simulink model "trajectory"  (R2021a)
settings: Solver=VariableStepAuto  StartTime=0.0  StopTime=10.0  RelTol=1e-3
libraries: robotcorelib x2
settings Model: Creator=ASUS  LastModifiedBy=ASUS

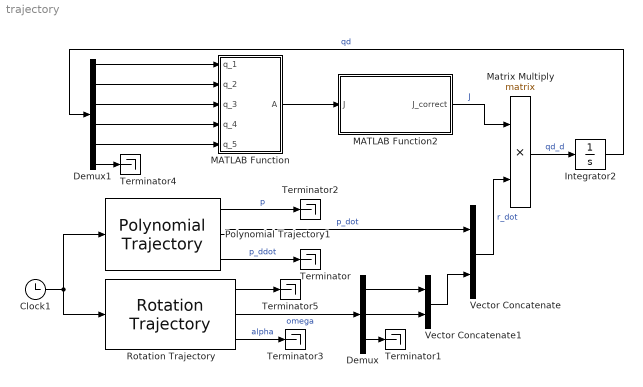
== system trajectory ==
  Clock1 : Clock
  Demux : Demux  Outputs=3
  Demux1 : Demux  Outputs=6
  Integrator2 : Integrator  InitialCondition=2
  MATLAB Function : MATLAB Function  TreatAsAtomicUnit=on
  MATLAB Function2 : MATLAB Function  TreatAsAtomicUnit=on
  Matrix Multiply : Product  Multiplication=Matrix(*)
  Polynomial Trajectory1 : robotcorelib/Polynomial Trajectory  WaypointSource=Internal  Waypoints=[ 0, 0.1, 0.1; 0, 0.2, 0.1; 0, 0.1, 0.1]  TimePoints=[ 0, 3, 5 ]  TimeInterval=[ 1, 4 ]  Method=Cubic Polynomial  ParameterSource=Internal  VelocityBoundaryCondition=zeros( 3, 3)  AccelerationBoundaryCondition=zeros( 2, 5 )  SimulateUsing=Interpreted execution
  Rotation Trajectory : robotcorelib/Rotation Trajectory  WaypointFormat=Quaternion  WaypointSource=Internal  R0=[ 1, 0, 0, 0 ]'  RF=[ 0.1, 0.2, 0.5, 0 ]'  TimeInterval=[ 0, 5 ]  CustomTimeScaling=off  ParameterSource=Internal  TSTime=0:0.1:1  TimeScaling=[ 0:0.1:1; ones( 1, 11 ); zeros( 1, 11 ) ]  SimulateUsing=Interpreted execution
      settings: SourceProductBaseCode=NV,RO,RR,UV
  Terminator{,1..5} (6 alike) : Terminator
  Vector Concatenate : Concatenate
  Vector Concatenate1 : Concatenate
  wires:
  Clock1/1 -> Polynomial Trajectory1/1, Rotation Trajectory/1
  Polynomial Trajectory1/3 -> Terminator/1  "p_ddot"
  Polynomial Trajectory1/2 -> Vector Concatenate/1  "p_dot"
  Polynomial Trajectory1/1 -> Terminator2/1  "p"
  Rotation Trajectory/1 -> Terminator5/1
  Rotation Trajectory/3 -> Terminator3/1  "alpha"
  MATLAB Function/1(A) -> MATLAB Function2/1(J)
  MATLAB Function2/1(J_correct) -> Matrix Multiply/1  "J"
  Demux/3 -> Terminator1/1
  Demux/1 -> Vector Concatenate1/1
  Demux/2 -> Vector Concatenate1/2
  Rotation Trajectory/2 -> Demux/1  "omega"
  Vector Concatenate1/1 -> Vector Concatenate/2
  Vector Concatenate/1 -> Matrix Multiply/2  "r_dot"
  Matrix Multiply/1 -> Integrator2/1  "qd_d"
  Integrator2/1 -> Demux1/1  "qd"
  Demux1/6 -> Terminator4/1
  Demux1/1 -> MATLAB Function/1(q_1)
  Demux1/2 -> MATLAB Function/2(q_2)
  Demux1/3 -> MATLAB Function/3(q_3)
  Demux1/4 -> MATLAB Function/4(q_4)
  Demux1/5 -> MATLAB Function/5(q_5)

== matlab function trajectory/MATLAB Function ==
  data: q_1 input; A output; q_2 input; q_3 input; q_4 input; q_5 input
function A = fcn(q_1,q_2,q_3,q_4,q_5)


A = reshape([cos(q_1).*(cos(q_5).*8.1141e-2-cos(q_1).*(cos(q_3).*(sin(q_4).*sin(q_5).*8.1141e-2-cos(q_4).*(cos(q_5).*4.968453296480769e-18-9.456e-2))+sin(q_3).*(cos(q_4).*sin(q_5).*8.1141e-2+sin(q_4).*(cos(q_5).*4.968453296480769e-18-9.456e-2)+3.9225e-1)).*6.123233995736766e-17-sin(q_2).*(cos(q_3).*(cos(q_4).*sin(q_5).*8.1141e-2+sin(q_4).*(cos(q_5).*4.968453296480769e-18-9.456e-2)+3.9225e-1)-sin(q_3).*(sin(q_4).*sin(q_5).*8.1141e-2-cos(q_4).*(cos(q_5).*4.968453296480769e-18-9.456e-2))+1.7e+1./4.0e+1).*6.123233995736766e-17+1.0915e-1)-sin(q_1).*(cos(q_2).*(cos(q_3).*(cos(q_4).*sin(q_5).*8.1141e-2+sin(q_4).*(cos(q_5).*4.968453296480769e-18-9.456e-2)+3.9225e-1)-sin(q_3).*(sin(q_4).*sin(q_5).*8.1141e-2-cos(q_4).*(cos(q_5).*4.968453296480769e-18-9.456e-2))+1.7e+1./4.0e+1)-sin(q_2).*(cos(q_3).*(sin(q_4).*sin(q_5).*8.1141e-2-cos(q_4).*(cos(q_5).*4.968453296480769e-18-9.456e-2))+sin(q_3).*(cos(q_4).*sin(q_5).*8.1141e-2+sin(q_4).*(cos(q_5).*4.968453296480769e-18-9.456e-2)+3.9225e-1)))+sin(q_1).^2.*(cos(q_3).*(sin(q_4).*sin(q_5).*8.1141e-2-cos(q_4).*(cos(q_5).*4.968453296480769e-18-9.456e-2))+sin(q_3).*(cos(q_4).*sin(q_5).*8.1141e-2+sin(q_4).*(cos(q_5).*4.968453296480769e-18-9.456e-2)+3.9225e-1)).*6.123233995736766e-17,sin(q_1).*(cos(q_5).*8.1141e-2-cos(q_1).*(cos(q_3).*(sin(q_4).*sin(q_5).*8.1141e-2-cos(q_4).*(cos(q_5).*4.968453296480769e-18-9.456e-2))+sin(q_3).*(cos(q_4).*sin(q_5).*8.1141e-2+sin(q_4).*(cos(q_5).*4.968453296480769e-18-9.456e-2)+3.9225e-1)).*6.123233995736766e-17-sin(q_2).*(cos(q_3).*(cos(q_4).*sin(q_5).*8.1141e-2+sin(q_4).*(cos(q_5).*4.968453296480769e-18-9.456e-2)+3.9225e-1)-sin(q_3).*(sin(q_4).*sin(q_5).*8.1141e-2-cos(q_4).*(cos(q_5).*4.968453296480769e-18-9.456e-2))+1.7e+1./4.0e+1).*6.123233995736766e-17+1.0915e-1)+cos(q_1).*(cos(q_2).*(cos(q_3).*(cos(q_4).*sin(q_5).*8.1141e-2+sin(q_4).*(cos(q_5).*4.968453296480769e-18-9.456e-2)+3.9225e-1)-sin(q_3).*(sin(q_4).*sin(q_5).*8.1141e-2-cos(q_4).*(cos(q_5).*4.968453296480769e-18-9.456e-2))+1.7e+1./4.0e+1)-sin(q_2).*(cos(q_3).*(sin(q_4).*sin(q_5).*8.1141e-2-cos(q_4).*(cos(q_5).*4.968453296480769e-18-9.456e-2))+sin(q_3).*(cos(q_4).*sin(q_5).*8.1141e-2+sin(q_4).*(cos(q_5).*4.968453296480769e-18-9.456e-2)+3.9225e-1)))-cos(q_1).*sin(q_1).*(cos(q_3).*(sin(q_4).*sin(q_5).*8.1141e-2-cos(q_4).*(cos(q_5).*4.968453296480769e-18-9.456e-2))+sin(q_3).*(cos(q_4).*sin(q_5).*8.1141e-2+sin(q_4).*(cos(q_5).*4.968453296480769e-18-9.456e-2)+3.9225e-1)).*6.123233995736766e-17,0.0,0.0,0.0,1.0,-cos(q_1).*(cos(q_2).*(cos(q_3).*(sin(q_4).*sin(q_5).*8.1141e-2-cos(q_4).*(cos(q_5).*4.968453296480769e-18-9.456e-2))+sin(q_3).*(cos(q_4).*sin(q_5).*8.1141e-2+sin(q_4).*(cos(q_5).*4.968453296480769e-18-9.456e-2)+3.9225e-1))+sin(q_2).*(cos(q_3).*(cos(q_4).*sin(q_5).*8.1141e-2+sin(q_4).*(cos(q_5).*4.968453296480769e-18-9.456e-2)+3.9225e-1)-sin(q_3).*(sin(q_4).*sin(q_5).*8.1141e-2-cos(q_4).*(cos(q_5).*4.968453296480769e-18-9.456e-2))+1.7e+1./4.0e+1))-cos(q_2).*sin(q_1).*(cos(q_3).*(cos(q_4).*sin(q_5).*8.1141e-2+sin(q_4).*(cos(q_5).*4.968453296480769e-18-9.456e-2)+3.9225e-1)-sin(q_3).*(sin(q_4).*sin(q_5).*8.1141e-2-cos(q_4).*(cos(q_5).*4.968453296480769e-18-9.456e-2))+1.7e+1./4.0e+1).*6.123233995736766e-17,-sin(q_1).*(cos(q_2).*(cos(q_3).*(sin(q_4).*sin(q_5).*8.1141e-2-cos(q_4).*(cos(q_5).*4.968453296480769e-18-9.456e-2))+sin(q_3).*(cos(q_4).*sin(q_5).*8.1141e-2+sin(q_4).*(cos(q_5).*4.968453296480769e-18-9.456e-2)+3.9225e-1))+sin(q_2).*(cos(q_3).*(cos(q_4).*sin(q_5).*8.1141e-2+sin(q_4).*(cos(q_5).*4.968453296480769e-18-9.456e-2)+3.9225e-1)-sin(q_3).*(sin(q_4).*sin(q_5).*8.1141e-2-cos(q_4).*(cos(q_5).*4.968453296480769e-18-9.456e-2))+1.7e+1./4.0e+1))+cos(q_1).*cos(q_2).*(cos(q_3).*(cos(q_4).*sin(q_5).*8.1141e-2+sin(q_4).*(cos(q_5).*4.968453296480769e-18-9.456e-2)+3.9225e-1)-sin(q_3).*(sin(q_4).*sin(q_5).*8.1141e-2-cos(q_4).*(cos(q_5).*4.968453296480769e-18-9.456e-2))+1.7e+1./4.0e+1).*6.123233995736766e-17,cos(q_2).*(cos(q_3).*(cos(q_4).*sin(q_5).*8.1141e-2+sin(q_4).*(cos(q_5).*4.968453296480769e-18-9.456e-2)+3.9225e-1)-sin(q_3).*(sin(q_4).*sin(q_5).*8.1141e-2-cos(q_4).*(cos(q_5).*4.968453296480769e-18-9.456e-2))+1.7e+1./4.0e+1)-sin(q_2).*(cos(q_3).*(sin(q_4).*sin(q_5).*8.1141e-2-cos(q_4).*(cos(q_5).*4.968453296480769e-18-9.456e-2))+sin(q_3).*(cos(q_4).*sin(q_5).*8.1141e-2+sin(q_4).*(cos(q_5).*4.968453296480769e-18-9.456e-2)+3.9225e-1)),sin(q_1),-cos(q_1),6.123233995736766e-17,-cos(q_1).*(cos(q_2).*(cos(q_3).*(sin(q_4).*sin(q_5).*8.1141e-2-cos(q_4).*(cos(q_5).*4.968453296480769e-18-9.456e-2))+sin(q_3).*(cos(q_4).*sin(q_5).*8.1141e-2+sin(q_4).*(cos(q_5).*4.968453296480769e-18-9.456e-2)+3.9225e-1))+sin(q_2).*(cos(q_3).*(cos(q_4).*sin(q_5).*8.1141e-2+sin(q_4).*(cos(q_5).*4.968453296480769e-18-9.456e-2)+3.9225e-1)-sin(q_3).*(sin(q_4).*sin(q_5).*8.1141e-2-cos(q_4).*(cos(q_5).*4.968453296480769e-18-9.456e-2))))-sin(q_1).*(cos(q_1).*(cos(q_3).*(cos(q_4).*sin(q_5).*8.1141e-2+sin(q_4).*(cos(q_5).*4.968453296480769e-18-9.456e-2)+3.9225e-1)-sin(q_3).*(sin(q_4).*sin(q_5).*8.1141e-2-cos(q_4).*(cos(q_5).*4.968453296480769e-18-9.456e-2))).*6.123233995736766e-17-sin(q_2).*(cos(q_3).*(sin(q_4).*sin(q_5).*8.1141e-2-cos(q_4).*(cos(q_5).*4.968453296480769e-18-9.456e-2))+sin(q_3).*(cos(q_4).*sin(q_5).*8.1141e-2+sin(q_4).*(cos(q_5).*4.968453296480769e-18-9.456e-2)+3.9225e-1)).*6.123233995736766e-17),-sin(q_1).*(cos(q_2).*(cos(q_3).*(sin(q_4).*sin(q_5).*8.1141e-2-cos(q_4).*(cos(q_5).*4.968453296480769e-18-9.456e-2))+sin(q_3).*(cos(q_4).*sin(q_5).*8.1141e-2+sin(q_4).*(cos(q_5).*4.968453296480769e-18-9.456e-2)+3.9225e-1))+sin(q_2).*(cos(q_3).*(cos(q_4).*sin(q_5).*8.1141e-2+sin(q_4).*(cos(q_5).*4.968453296480769e-18-9.456e-2)+3.9225e-1)-sin(q_3).*(sin(q_4).*sin(q_5).*8.1141e-2-cos(q_4).*(cos(q_5).*4.968453296480769e-18-9.456e-2))))+cos(q_1).*(cos(q_1).*(cos(q_3).*(cos(q_4).*sin(q_5).*8.1141e-2+sin(q_4).*(cos(q_5).*4.968453296480769e-18-9.456e-2)+3.9225e-1)-sin(q_3).*(sin(q_4).*sin(q_5).*8.1141e-2-cos(q_4).*(cos(q_5).*4.968453296480769e-18-9.456e-2))).*6.123233995736766e-17-sin(q_2).*(cos(q_3).*(sin(q_4).*sin(q_5).*8.1141e-2-cos(q_4).*(cos(q_5).*4.968453296480769e-18-9.456e-2))+sin(q_3).*(cos(q_4).*sin(q_5).*8.1141e-2+sin(q_4).*(cos(q_5).*4.968453296480769e-18-9.456e-2)+3.9225e-1)).*6.123233995736766e-17),cos(q_2).*(cos(q_3).*(cos(q_4).*sin(q_5).*8.1141e-2+sin(q_4).*(cos(q_5).*4.968453296480769e-18-9.456e-2)+3.9225e-1)-sin(q_3).*(sin(q_4).*sin(q_5).*8.1141e-2-cos(q_4).*(cos(q_5).*4.968453296480769e-18-9.456e-2)))-sin(q_2).*(cos(q_3).*(sin(q_4).*sin(q_5).*8.1141e-2-cos(q_4).*(cos(q_5).*4.968453296480769e-18-9.456e-2))+sin(q_3).*(cos(q_4).*sin(q_5).*8.1141e-2+sin(q_4).*(cos(q_5).*4.968453296480769e-18-9.456e-2)+3.9225e-1)),sin(q_1),-cos(q_1),6.123233995736766e-17,-cos(q_1).*(cos(q_2).*(cos(q_3).*(sin(q_4).*sin(q_5).*8.1141e-2-cos(q_4).*(cos(q_5).*4.968453296480769e-18-9.456e-2))+sin(q_3).*(cos(q_4).*sin(q_5).*8.1141e-2+sin(q_4).*(cos(q_5).*4.968453296480769e-18-9.456e-2)))+sin(q_2).*(cos(q_3).*(cos(q_4).*sin(q_5).*8.1141e-2+sin(q_4).*(cos(q_5).*4.968453296480769e-18-9.456e-2))-sin(q_3).*(sin(q_4).*sin(q_5).*8.1141e-2-cos(q_4).*(cos(q_5).*4.968453296480769e-18-9.456e-2))))-sin(q_1).*(cos(q_1).*(cos(q_3).*(cos(q_4).*sin(q_5).*8.1141e-2+sin(q_4).*(cos(q_5).*4.968453296480769e-18-9.456e-2))-sin(q_3).*(sin(q_4).*sin(q_5).*8.1141e-2-cos(q_4).*(cos(q_5).*4.968453296480769e-18-9.456e-2))).*6.123233995736766e-17-sin(q_2).*(cos(q_3).*(sin(q_4).*sin(q_5).*8.1141e-2-cos(q_4).*(cos(q_5).*4.968453296480769e-18-9.456e-2))+sin(q_3).*(cos(q_4).*sin(q_5).*8.1141e-2+sin(q_4).*(cos(q_5).*4.968453296480769e-18-9.456e-2))).*6.123233995736766e-17),-sin(q_1).*(cos(q_2).*(cos(q_3).*(sin(q_4).*sin(q_5).*8.1141e-2-cos(q_4).*(cos(q_5).*4.968453296480769e-18-9.456e-2))+sin(q_3).*(cos(q_4).*sin(q_5).*8.1141e-2+sin(q_4).*(cos(q_5).*4.968453296480769e-18-9.456e-2)))+sin(q_2).*(cos(q_3).*(cos(q_4).*sin(q_5).*8.1141e-2+sin(q_4).*(cos(q_5).*4.968453296480769e-18-9.456e-2))-sin(q_3).*(sin(q_4).*sin(q_5).*8.1141e-2-cos(q_4).*(cos(q_5).*4.968453296480769e-18-9.456e-2))))+cos(q_1).*(cos(q_1).*(cos(q_3).*(cos(q_4).*sin(q_5).*8.1141e-2+sin(q_4).*(cos(q_5).*4.968453296480769e-18-9.456e-2))-sin(q_3).*(sin(q_4).*sin(q_5).*8.1141e-2-cos(q_4).*(cos(q_5).*4.968453296480769e-18-9.456e-2))).*6.123233995736766e-17-sin(q_2).*(cos(q_3).*(sin(q_4).*sin(q_5).*8.1141e-2-cos(q_4).*(cos(q_5).*4.968453296480769e-18-9.456e-2))+sin(q_3).*(cos(q_4).*sin(q_5).*8.1141e-2+sin(q_4).*(cos(q_5).*4.968453296480769e-18-9.456e-2))).*6.123233995736766e-17),cos(q_2).*(cos(q_3).*(cos(q_4).*sin(q_5).*8.1141e-2+sin(q_4).*(cos(q_5).*4.968453296480769e-18-9.456e-2))-sin(q_3).*(sin(q_4).*sin(q_5).*8.1141e-2-cos(q_4).*(cos(q_5).*4.968453296480769e-18-9.456e-2)))-sin(q_2).*(cos(q_3).*(sin(q_4).*sin(q_5).*8.1141e-2-cos(q_4).*(cos(q_5).*4.968453296480769e-18-9.456e-2))+sin(q_3).*(cos(q_4).*sin(q_5).*8.1141e-2+sin(q_4).*(cos(q_5).*4.968453296480769e-18-9.456e-2))),sin(q_1),-cos(q_1),6.123233995736766e-17,cos(q_1).*(cos(q_2).*(cos(q_3).*(cos(q_4).*cos(q_5).*8.1141e-2-sin(q_4).*sin(q_5).*4.968453296480769e-18)-sin(q_3).*(cos(q_4).*sin(q_5).*4.968453296480769e-18+cos(q_5).*sin(q_4).*8.1141e-2))-sin(q_2).*(cos(q_3).*(cos(q_4).*sin(q_5).*4.968453296480769e-18+cos(q_5).*sin(q_4).*8.1141e-2)+sin(q_3).*(cos(q_4).*cos(q_5).*8.1141e-2-sin(q_4).*sin(q_5).*4.968453296480769e-18)))-sin(q_1).*(sin(q_5).*8.1141e-2+cos(q_1).*(cos(q_3).*(cos(q_4).*sin(q_5).*4.968453296480769e-18+cos(q_5).*sin(q_4).*8.1141e-2)+sin(q_3).*(cos(q_4).*cos(q_5).*8.1141e-2-sin(q_4).*sin(q_5).*4.968453296480769e-18)).*6.123233995736766e-17+sin(q_2).*(cos(q_3).*(cos(q_4).*cos(q_5).*8.1141e-2-sin(q_4).*sin(q_5).*4.968453296480769e-18)-sin(q_3).*(cos(q_4).*sin(q_5).*4.968453296480769e-18+cos(q_5).*sin(q_4).*8.1141e-2)).*6.123233995736766e-17),sin(q_1).*(cos(q_2).*(cos(q_3).*(cos(q_4).*cos(q_5).*8.1141e-2-sin(q_4).*sin(q_5).*4.968453296480769e-18)-sin(q_3).*(cos(q_4).*sin(q_5).*4.968453296480769e-18+cos(q_5).*sin(q_4).*8.1141e-2))-sin(q_2).*(cos(q_3).*(cos(q_4).*sin(q_5).*4.968453296480769e-18+cos(q_5).*sin(q_4).*8.1141e-2)+sin(q_3).*(cos(q_4).*cos(q_5).*8.1141e-2-sin(q_4).*sin(q_5).*4.968453296480769e-18)))+cos(q_1).*(sin(q_5).*8.1141e-2+cos(q_1).*(cos(q_3).*(cos(q_4).*sin(q_5).*4.968453296480769e-18+cos(q_5).*sin(q_4).*8.1141e-2)+sin(q_3).*(cos(q_4).*cos(q_5).*8.1141e-2-sin(q_4).*sin(q_5).*4.968453296480769e-18)).*6.123233995736766e-17+sin(q_2).*(cos(q_3).*(cos(q_4).*cos(q_5).*8.1141e-2-sin(q_4).*sin(q_5).*4.968453296480769e-18)-sin(q_3).*(cos(q_4).*sin(q_5).*4.968453296480769e-18+cos(q_5).*sin(q_4).*8.1141e-2)).*6.123233995736766e-17),sin(q_5).*(-4.968453296480769e-18)+cos(q_2).*(cos(q_3).*(cos(q_4).*sin(q_5).*4.968453296480769e-18+cos(q_5).*sin(q_4).*8.1141e-2)+sin(q_3).*(cos(q_4).*cos(q_5).*8.1141e-2-sin(q_4).*sin(q_5).*4.968453296480769e-18))+sin(q_2).*(cos(q_3).*(cos(q_4).*cos(q_5).*8.1141e-2-sin(q_4).*sin(q_5).*4.968453296480769e-18)-sin(q_3).*(cos(q_4).*sin(q_5).*4.968453296480769e-18+cos(q_5).*sin(q_4).*8.1141e-2)),sin(q_1).*6.123233995736766e-17-cos(q_4).*(sin(q_3).*(cos(q_1).*cos(q_2)-sin(q_1).*sin(q_2).*6.123233995736766e-17)+cos(q_3).*(cos(q_1).*sin(q_1).*6.123233995736766e-17+cos(q_1).*sin(q_2)))+sin(q_4).*(sin(q_3).*(cos(q_1).*sin(q_1).*6.123233995736766e-17+cos(q_1).*sin(q_2))-cos(q_3).*(cos(q_1).*cos(q_2)-sin(q_1).*sin(q_2).*6.123233995736766e-17)),cos(q_1).*(-6.123233995736766e-17)-cos(q_4).*(sin(q_3).*(cos(q_1).*sin(q_2).*6.123233995736766e-17+cos(q_2).*sin(q_1))+cos(q_3).*(sin(q_1).*sin(q_2)-cos(q_1).^2.*6.123233995736766e-17))+sin(q_4).*(sin(q_3).*(sin(q_1).*sin(q_2)-cos(q_1).^2.*6.123233995736766e-17)-cos(q_3).*(cos(q_1).*sin(q_2).*6.123233995736766e-17+cos(q_2).*sin(q_1))),cos(q_4).*(cos(q_2).*cos(q_3)-sin(q_2).*sin(q_3))-sin(q_4).*(cos(q_2).*sin(q_3)+cos(q_3).*sin(q_2))+3.749399456654644e-33,0.0,0.0,0.0,sin(q_1).*3.749399456654644e-33+cos(q_5).*sin(q_1)-cos(q_4).*(sin(q_3).*(cos(q_1).*cos(q_2)-sin(q_1).*sin(q_2).*6.123233995736766e-17)+cos(q_3).*(cos(q_1).*sin(q_1).*6.123233995736766e-17+cos(q_1).*sin(q_2))).*6.123233995736766e-17+sin(q_4).*(sin(q_3).*(cos(q_1).*sin(q_1).*6.123233995736766e-17+cos(q_1).*sin(q_2))-cos(q_3).*(cos(q_1).*cos(q_2)-sin(q_1).*sin(q_2).*6.123233995736766e-17)).*6.123233995736766e-17+cos(q_5).*(cos(q_4).*(sin(q_3).*(cos(q_1).*cos(q_2)-sin(q_1).*sin(q_2).*6.123233995736766e-17)+cos(q_3).*(cos(q_1).*sin(q_1).*6.123233995736766e-17+cos(q_1).*sin(q_2)))-sin(q_4).*(sin(q_3).*(cos(q_1).*sin(q_1).*6.123233995736766e-17+cos(q_1).*sin(q_2))-cos(q_3).*(cos(q_1).*cos(q_2)-sin(q_1).*sin(q_2).*6.123233995736766e-17))).*6.123233995736766e-17-sin(q_5).*(cos(q_4).*(sin(q_3).*(cos(q_1).*sin(q_1).*6.123233995736766e-17+cos(q_1).*sin(q_2))-cos(q_3).*(cos(q_1).*cos(q_2)-sin(q_1).*sin(q_2).*6.123233995736766e-17))+sin(q_4).*(sin(q_3).*(cos(q_1).*cos(q_2)-sin(q_1).*sin(q_2).*6.123233995736766e-17)+cos(q_3).*(cos(q_1).*sin(q_1).*6.123233995736766e-17+cos(q_1).*sin(q_2)))),cos(q_1).*(-3.749399456654644e-33)-cos(q_1).*cos(q_5)-cos(q_4).*(sin(q_3).*(cos(q_1).*sin(q_2).*6.123233995736766e-17+cos(q_2).*sin(q_1))+cos(q_3).*(sin(q_1).*sin(q_2)-cos(q_1).^2.*6.123233995736766e-17)).*6.123233995736766e-17+sin(q_4).*(sin(q_3).*(sin(q_1).*sin(q_2)-cos(q_1).^2.*6.123233995736766e-17)-cos(q_3).*(cos(q_1).*sin(q_2).*6.123233995736766e-17+cos(q_2).*sin(q_1))).*6.123233995736766e-17+cos(q_5).*(cos(q_4).*(sin(q_3).*(cos(q_1).*sin(q_2).*6.123233995736766e-17+cos(q_2).*sin(q_1))+cos(q_3).*(sin(q_1).*sin(q_2)-cos(q_1).^2.*6.123233995736766e-17))-sin(q_4).*(sin(q_3).*(sin(q_1).*sin(q_2)-cos(q_1).^2.*6.123233995736766e-17)-cos(q_3).*(cos(q_1).*sin(q_2).*6.123233995736766e-17+cos(q_2).*sin(q_1)))).*6.123233995736766e-17-sin(q_5).*(cos(q_4).*(sin(q_3).*(sin(q_1).*sin(q_2)-cos(q_1).^2.*6.123233995736766e-17)-cos(q_3).*(cos(q_1).*sin(q_2).*6.123233995736766e-17+cos(q_2).*sin(q_1)))+sin(q_4).*(sin(q_3).*(cos(q_1).*sin(q_2).*6.123233995736766e-17+cos(q_2).*sin(q_1))+cos(q_3).*(sin(q_1).*sin(q_2)-cos(q_1).^2.*6.123233995736766e-17))),cos(q_5).*6.123233995736766e-17-cos(q_5).*(cos(q_4).*(cos(q_2).*cos(q_3)-sin(q_2).*sin(q_3))-sin(q_4).*(cos(q_2).*sin(q_3)+cos(q_3).*sin(q_2))).*6.123233995736766e-17+sin(q_5).*(cos(q_4).*(cos(q_2).*sin(q_3)+cos(q_3).*sin(q_2))+sin(q_4).*(cos(q_2).*cos(q_3)-sin(q_2).*sin(q_3)))+cos(q_4).*(cos(q_2).*cos(q_3)-sin(q_2).*sin(q_3)).*6.123233995736766e-17-sin(q_4).*(cos(q_2).*sin(q_3)+cos(q_3).*sin(q_2)).*6.123233995736766e-17+2.295845021658468e-49],[6,6]);


end

== matlab function trajectory/MATLAB Function2 ==
  data: J input; J_correct output
function J_correct = fcn(J)

mu = 2;
J = J(1:5,:);
J_correct = J'/(J*J'+mu*eye(size(J,1)));

end
